simulink model "for_report"  (R2025b)
settings: Solver=VariableStepAuto  StartTime=0.0  StopTime=10.0  RelTol=1e-3
undefined symbols (not defined in the file): A_eqv, index, Jsum, k_feedforward, kc, kci, kdc, kds, ke, km, kp, ks, ksi, Kspr, Mext, omega_eqv, Ra, Te, Tsh
libraries: simulink x1
settings Model: Creator=Lenovo  LastModifiedBy=Lenovo

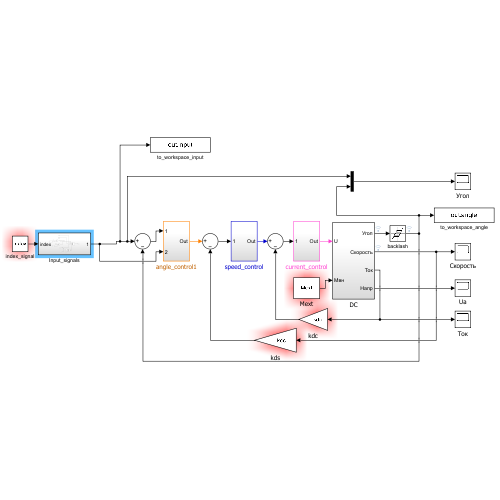
[thumbnail: Simulink's stored preview of the top-level diagram]
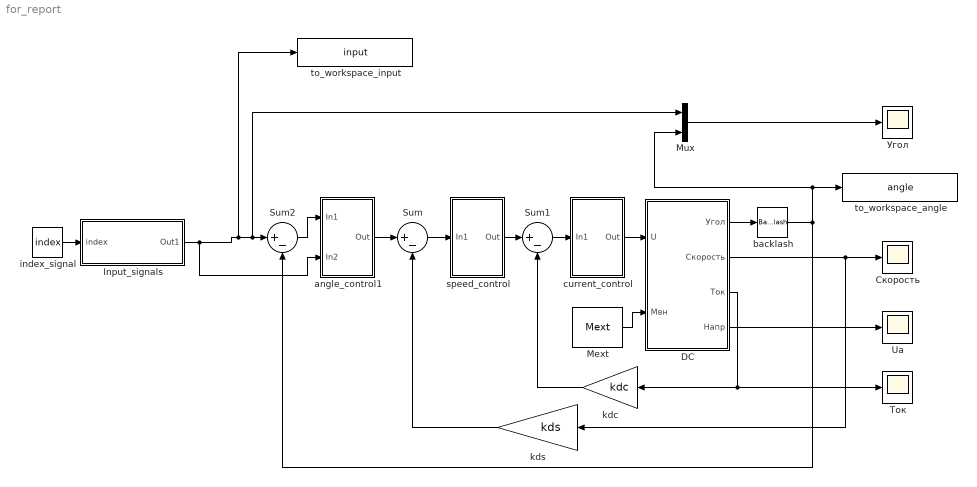
== system for_report ==
  DC : Subsystem
  Input_signals : Subsystem
  Mext : Constant  Value=Mext
  Mux : Mux  Inputs=2
  Sum : Sum  Inputs=|+-  SaturateOnIntegerOverflow=on
  Sum1 : Sum  Inputs=|+-  SaturateOnIntegerOverflow=on
  Sum2 : Sum  Inputs=|+-  SaturateOnIntegerOverflow=on
  Ua : Scope
      settings: SampleTime=0.001  TimeSpan=0.05353611419143481  ActiveDisplayYMinimum=-29.029207995662105  ActiveDisplayYMaximum=21.262871960959007  DataLoggingMaxPoints=50000  DataLoggingVariableName=ScopeData3
  angle_control1 : Subsystem
  backlash : Backlash  BacklashWidth=0.00015
  current_control : Subsystem
  index_signal : Constant  Value=index
  kdc : Gain  Gain=kdc  SaturateOnIntegerOverflow=on  OutDataTypeStr=Inherit: Same as input  ParamDataTypeStr=Inherit: Same as input
  kds : Gain  Gain=kds  SaturateOnIntegerOverflow=on  OutDataTypeStr=Inherit: Same as input  ParamDataTypeStr=Inherit: Same as input
  speed_control : Subsystem
  to_workspace_angle : ToWorkspace  VariableName=angle  SaveFormat=Structure With Time  SampleTime=-1
  to_workspace_input : ToWorkspace  VariableName=input  SaveFormat=Structure With Time  SampleTime=-1
  Скорость : Scope
      settings: ActiveDisplayYMinimum=-1.8818916422998546  ActiveDisplayYMaximum=14.765924340526233  DataLoggingMaxPoints=50000
  Ток : Scope
      settings: SampleTime=0.00001  TimeSpan=0.5  ActiveDisplayYMinimum=-1.8277716074712291  ActiveDisplayYMaximum=16.449944467241068  DataLoggingMaxPoints=50000  DataLoggingVariableName=ScopeData2
  Угол : Scope
      settings: SampleTime=0.001  ActiveDisplayYMinimum=-0.12499999999999997  ActiveDisplayYMaximum=1.125  DataLoggingMaxPoints=50000  DataLoggingVariableName=ScopeData8
  wires:
  Input_signals/1(Out1) -> angle_control1/2(In2), Mux/1, Sum2/1, to_workspace_input/1
  DC/1(Угол) -> backlash/1
  DC/2(Скорость) -> kds/1, Скорость/1
  Sum2/1 -> angle_control1/1(In1)
  speed_control/1(Out) -> Sum1/1
  kds/1 -> Sum/2
  backlash/1 -> Mux/2, to_workspace_angle/1, Sum2/2
  Mext/1 -> DC/2(Mвн)
  Sum/1 -> speed_control/1(In1)
  DC/4(Напр) -> Ua/1
  current_control/1(Out) -> DC/1(U)
  DC/3(Ток) -> Ток/1, kdc/1
  kdc/1 -> Sum1/2
  index_signal/1 -> Input_signals/1(index)
  Sum1/1 -> current_control/1(In1)
  angle_control1/1(Out) -> Sum/1
  Mux/1 -> Угол/1

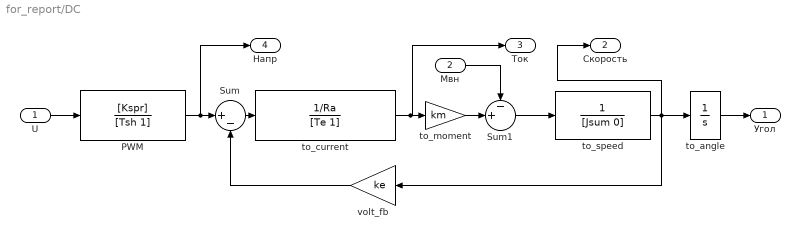
== system for_report/DC ==
  U : Inport
  Mвн : Inport  Port=2
  PWM : TransferFcn  Numerator=[Kspr]  Denominator=[Tsh 1]
  Sum : Sum  Inputs=|+-  InputSameDT=on  SaturateOnIntegerOverflow=on  OutDataTypeStr=Inherit: Same as first input
  Sum1 : Sum  Inputs=-+|  InputSameDT=on  SaturateOnIntegerOverflow=on  OutDataTypeStr=Inherit: Same as first input
  to_angle : Integrator
  to_current : TransferFcn  Numerator=1/Ra  Denominator=[Te 1]
  to_moment : Gain  Gain=km  SaturateOnIntegerOverflow=on  OutDataTypeStr=Inherit: Same as input  ParamDataTypeStr=Inherit: Same as input
  to_speed : TransferFcn  Denominator=[Jsum 0]
  volt_fb : Gain  Gain=ke  SaturateOnIntegerOverflow=on  OutDataTypeStr=Inherit: Same as input  ParamDataTypeStr=Inherit: Same as input
  Угол : Outport
  Скорость : Outport  Port=2
  Ток : Outport  Port=3
  Напр : Outport  Port=4
  wires:
  Mвн/1 -> Sum1/1
  Sum1/1 -> to_speed/1
  to_speed/1 -> volt_fb/1, Скорость/1, to_angle/1
  to_moment/1 -> Sum1/2
  to_angle/1 -> Угол/1
  U/1 -> PWM/1
  volt_fb/1 -> Sum/2
  to_current/1 -> Ток/1, to_moment/1
  PWM/1 -> Напр/1, Sum/1
  Sum/1 -> to_current/1

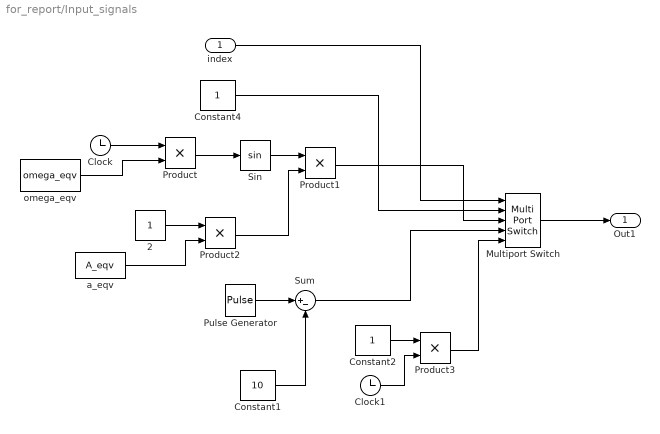
== system for_report/Input_signals ==
  index : Inport
  2 : Constant
  Clock : Clock
  Clock1 : Clock
  Constant1 : Constant  Value=10
  Constant2 : Constant
  Constant4 : Constant
  Multiport Switch : MultiPortSwitch  Inputs=4  SaturateOnIntegerOverflow=off  InputSameDT=off
  Product{,1..3} (4 alike) : Product
  Pulse Generator : DiscretePulseGenerator  PulseType=Time based  Amplitude=20  Period=1.5  PulseWidth=50
  Sin : Trigonometry
  Sum : Sum  Inputs=|+-
  a_eqv : Constant  Value=A_eqv
  omega_eqv : Constant  Value=omega_eqv
  Out1 : Outport
  wires:
  2/1 -> Product2/1
  Product/1 -> Sin/1
  Product2/1 -> Product1/2
  Clock/1 -> Product/1
  omega_eqv/1 -> Product/2
  Sin/1 -> Product1/1
  Constant2/1 -> Product3/1
  a_eqv/1 -> Product2/2
  Clock1/1 -> Product3/2
  Multiport Switch/1 -> Out1/1
  index/1 -> Multiport Switch/1
  Constant4/1 -> Multiport Switch/2
  Product1/1 -> Multiport Switch/3
  Pulse Generator/1 -> Sum/1
  Constant1/1 -> Sum/2
  Sum/1 -> Multiport Switch/4
  Product3/1 -> Multiport Switch/5

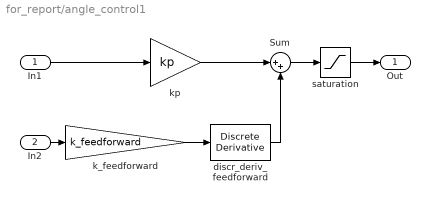
== system for_report/angle_control1 ==
  In1 : Inport
  In2 : Inport  Port=2
  Sum : Sum  Inputs=|++
  discr_deriv_feedforward : simulink/Quick Insert/Discrete/Discrete Derivative  gainval=1  ICPrevScaledInput=0.01  OutMin=[]  OutMax=[]  OutDataType=fixdt(1, 16)  OutScaling=2^-10  DoSatur=off
  k_feedforward : Gain  Gain=k_feedforward
  kp : Gain  Gain=kp  SaturateOnIntegerOverflow=on  OutDataTypeStr=Inherit: Same as input  ParamDataTypeStr=Inherit: Same as input
  saturation : Saturate  UpperLimit=10  LowerLimit=-10
  Out : Outport
  wires:
  saturation/1 -> Out/1
  kp/1 -> Sum/1
  Sum/1 -> saturation/1
  k_feedforward/1 -> discr_deriv_feedforward/1
  In2/1 -> k_feedforward/1
  discr_deriv_feedforward/1 -> Sum/2
  In1/1 -> kp/1

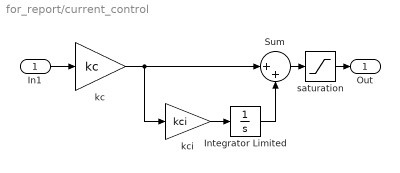
== system for_report/current_control ==
  In1 : Inport
  Integrator Limited : Integrator  LimitOutput=on  UpperSaturationLimit=10  LowerSaturationLimit=-10
  Sum : Sum  Inputs=|++  SaturateOnIntegerOverflow=on
  kc : Gain  Gain=kc  SaturateOnIntegerOverflow=on  OutDataTypeStr=Inherit: Same as input  ParamDataTypeStr=Inherit: Same as input
  kci : Gain  Gain=kci  SaturateOnIntegerOverflow=on  OutDataTypeStr=Inherit: Same as input  ParamDataTypeStr=Inherit: Same as input
  saturation : Saturate  UpperLimit=10  LowerLimit=-10
  Out : Outport
  wires:
  In1/1 -> kc/1
  kci/1 -> Integrator Limited/1
  Integrator Limited/1 -> Sum/2
  kc/1 -> Sum/1, kci/1
  Sum/1 -> saturation/1
  saturation/1 -> Out/1

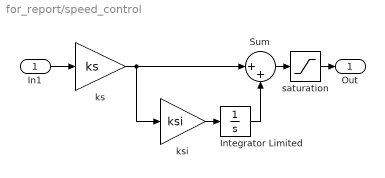
== system for_report/speed_control ==
  In1 : Inport
  Integrator Limited : Integrator  LimitOutput=on  UpperSaturationLimit=10  LowerSaturationLimit=-10
  Sum : Sum  Inputs=|++  SaturateOnIntegerOverflow=on
  ks : Gain  Gain=ks  SaturateOnIntegerOverflow=on  OutDataTypeStr=Inherit: Same as input  ParamDataTypeStr=Inherit: Same as input
  ksi : Gain  Gain=ksi  SaturateOnIntegerOverflow=on  OutDataTypeStr=Inherit: Same as input  ParamDataTypeStr=Inherit: Same as input
  saturation : Saturate  UpperLimit=10  LowerLimit=-10
  Out : Outport
  wires:
  In1/1 -> ks/1
  ks/1 -> Sum/1, ksi/1
  Integrator Limited/1 -> Sum/2
  ksi/1 -> Integrator Limited/1
  Sum/1 -> saturation/1
  saturation/1 -> Out/1
